simulink library "rwa_assembly_torqueinput_lib"  (R2018b)
settings: Solver=VariableStepAuto  StartTime=0.0  StopTime=10.0  RelTol=1e-3
undefined symbols (not defined in the file): fswParams
libraries: rw_motor_torqueinput_lib x4
settings Model: Creator=Taylor  LastModifiedBy=colem

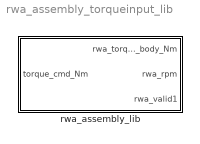
== system rwa_assembly_torqueinput_lib ==
  rwa_assembly_lib : Subsystem

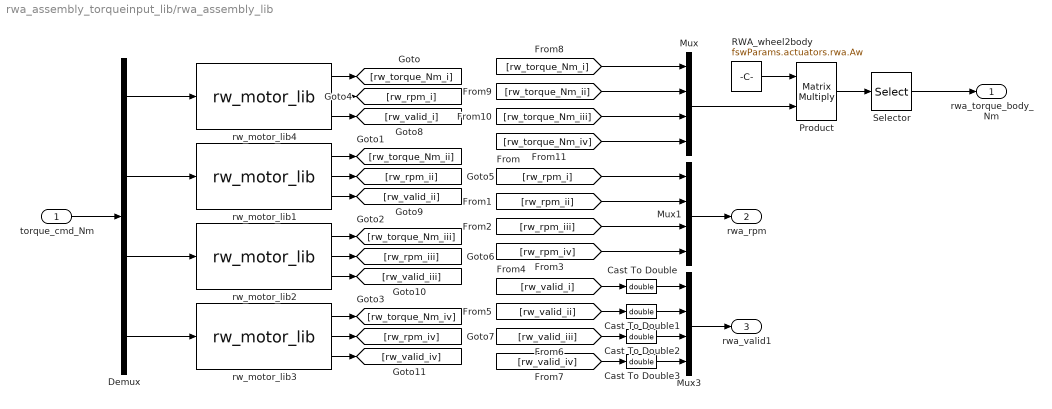
== system rwa_assembly_torqueinput_lib/rwa_assembly_lib ==
  torque_cmd_Nm : Inport
  Cast To Double{,1..3} (4 alike) : DataTypeConversion  OutDataTypeStr=double
  Demux : Demux
  Mux : Mux
  Mux1 : Mux
  Mux3 : Mux
  Product : Product  Multiplication=Matrix(*)
  RWA_wheel2body : Constant  Value=fswParams.actuators.rwa.Aw
  Selector : Selector  InputPortWidth=4  IndexOptions=Index vector (dialog)  Indices=[1 2 3]  OutputSizes=1
  rw_motor_lib1 : rw_motor_torqueinput_lib/rw_motor_lib  id_a=2
  rw_motor_lib2 : rw_motor_torqueinput_lib/rw_motor_lib  id_a=3
  rw_motor_lib3 : rw_motor_torqueinput_lib/rw_motor_lib  id_a=4
  rw_motor_lib4 : rw_motor_torqueinput_lib/rw_motor_lib  id_a=1
  rwa_torque_body_Nm : Outport
  rwa_rpm : Outport  Port=2
  rwa_valid1 : Outport  Port=3
  wires:
  torque_cmd_Nm/1 -> Demux/1
  Demux/1 -> rw_motor_lib4/1
  Demux/2 -> rw_motor_lib1/1
  Demux/3 -> rw_motor_lib2/1
  Demux/4 -> rw_motor_lib3/1
  rw_motor_lib4/1 -> [rw_torque_Nm_i]
  rw_motor_lib1/1 -> [rw_torque_Nm_ii]
  rw_motor_lib2/1 -> [rw_torque_Nm_iii]
  rw_motor_lib3/1 -> [rw_torque_Nm_iv]
  rw_motor_lib4/2 -> [rw_rpm_i]
  rw_motor_lib1/2 -> [rw_rpm_ii]
  rw_motor_lib2/2 -> [rw_rpm_iii]
  rw_motor_lib3/2 -> [rw_rpm_iv]
  Mux/1 -> Product/2
  Mux1/1 -> rwa_rpm/1
  [rw_rpm_i] -> Mux1/1
  [rw_rpm_ii] -> Mux1/2
  rw_motor_lib4/3 -> [rw_valid_i]
  rw_motor_lib1/3 -> [rw_valid_ii]
  rw_motor_lib2/3 -> [rw_valid_iii]
  rw_motor_lib3/3 -> [rw_valid_iv]
  [rw_rpm_iii] -> Mux1/3
  [rw_rpm_iv] -> Mux1/4
  Product/1 -> Selector/1
  [rw_torque_Nm_i] -> Mux/1
  [rw_torque_Nm_ii] -> Mux/2
  [rw_torque_Nm_iii] -> Mux/3
  [rw_torque_Nm_iv] -> Mux/4
  RWA_wheel2body/1 -> Product/1
  Selector/1 -> rwa_torque_body_Nm/1
  [rw_valid_i] -> Cast To Double/1
  [rw_valid_iii] -> Cast To Double2/1
  Cast To Double/1 -> Mux3/1
  Cast To Double1/1 -> Mux3/2
  [rw_valid_iv] -> Cast To Double3/1
  [rw_valid_ii] -> Cast To Double1/1
  Mux3/1 -> rwa_valid1/1
  Cast To Double3/1 -> Mux3/4
  Cast To Double2/1 -> Mux3/3
